simulink model "OpenDiscon_block"  (Simulink 10.1)
settings: Solver=ode45  StartTime=0.0  StopTime=10.0  RelTol=1e-3  EnableMultiTasking=on
settings Model: Creator=ielorza  LastModifiedBy=matlabktm1
settings DataIOCC: LimitDataPoints=on
settings DebuggingCC: UnderspecifiedInitializationDetection=Simplified  MergeDetectMultiDrivingBlocksExec=error  SolverPrmCheckMsg=warning
settings GRTTargetCC: CombineOutputUpdateFcns=on  GRTInterface=off
settings ConfigComp: CovSFcnEnable=off

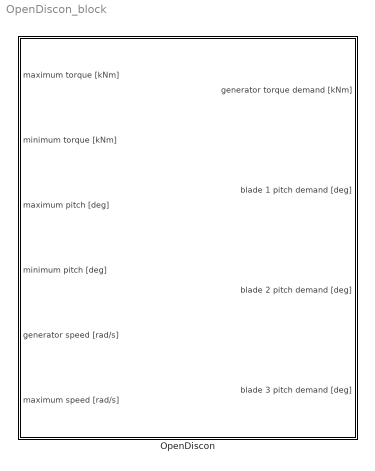
== system OpenDiscon_block ==
  OpenDiscon : Subsystem

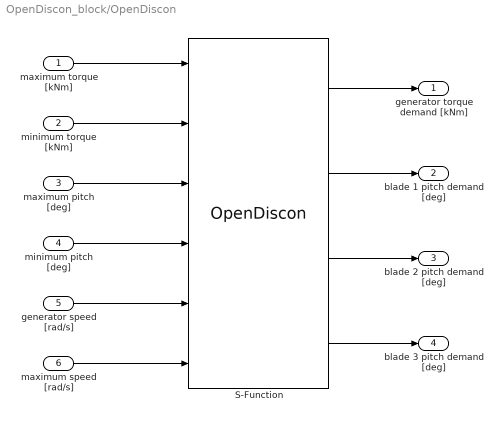
== system OpenDiscon_block/OpenDiscon ==
  maximum torque [kNm] : Inport
  minimum torque [kNm] : Inport  Port=2
  maximum pitch [deg] : Inport  Port=3
  minimum pitch [deg] : Inport  Port=4
  generator speed [rad/s] : Inport  Port=5
  maximum speed [rad/s] : Inport  Port=6
  S-Function : S-Function  FunctionName=OpenDiscon  SFunctionDeploymentMode=off  EnableBusSupport=off
  generator torque demand [kNm] : Outport
  blade 1 pitch demand [deg] : Outport  Port=2
  blade 2 pitch demand [deg] : Outport  Port=3
  blade 3 pitch demand [deg] : Outport  Port=4
  wires:
  maximum torque [kNm]/1 -> S-Function/1
  maximum pitch [deg]/1 -> S-Function/3
  minimum pitch [deg]/1 -> S-Function/4
  generator speed [rad/s]/1 -> S-Function/5
  minimum torque [kNm]/1 -> S-Function/2
  S-Function/4 -> blade 3 pitch demand [deg]/1
  S-Function/3 -> blade 2 pitch demand [deg]/1
  S-Function/2 -> blade 1 pitch demand [deg]/1
  S-Function/1 -> generator torque demand [kNm]/1
  maximum speed [rad/s]/1 -> S-Function/6
